simulink model "quadrotor_demo_xpc"  (Simulink 7.4)
settings: Solver=ode4  StartTime=0.0  StopTime=inf  FixedStep=0.01  RelTol=1e-3
libraries: xpcutilitieslib x23, aero_sim_lib x8, xpclib x2, simulink x1
settings Model: Creator=jporter  LastModifiedBy=jporter  SimulationMode=rapid-accelerator
settings SolverCC: AutoInsertRateTranBlk=on
settings DataIOCC: MaxDataPoints=5000  SaveFinalState=on  SaveState=on
settings OptimizationCC: InlineParams=on  EnhancedBackFolding=on  SimCompilerOptimization=On
settings HardwareCC: ProdIntDivRoundTo=Zero  ProdEndianess=LittleEndian  ProdHWDeviceType=Generic->32-bit x86 compatible
settings RTWCC: SystemTargetFile=xpctarget.tlc  TemplateMakefile=xpc_default_tmf  Description=xPC Target  ProcessScript=xpctarget_make_rtw_hook  RTWCompilerOptimization=On
settings xpcTargetCC: TargetFcnLib=ansi_tfl_table_tmw.mat  TargetFunctionLibrary=ANSI_C  ParMdlRefBuildCompliant=off  PortableWordSizes=off  xPCisDownloadable=off  xPCLoadParamSetFile=off

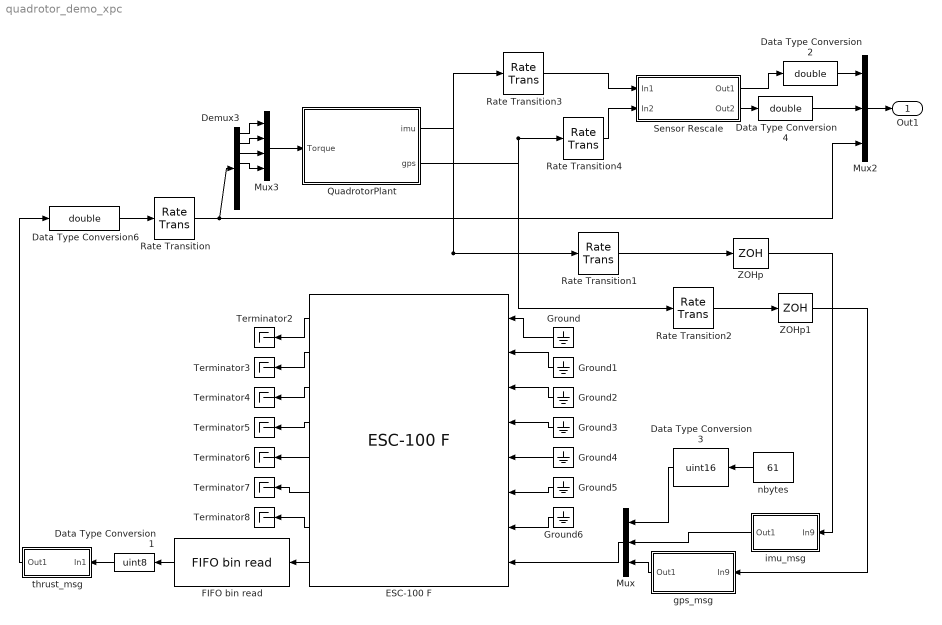
== system quadrotor_demo_xpc ==
  Data Type Conversion1 : DataTypeConversion  OutDataTypeMode=uint8  OutDataType=sfix(16)  OutScaling=2^0  OutDataTypeStr=uint8
  Data Type Conversion2 : DataTypeConversion  OutDataTypeMode=double  OutDataType=sfix(16)  OutScaling=2^0  OutDataTypeStr=double
  Data Type Conversion3 : DataTypeConversion  OutDataTypeMode=uint16  OutDataType=sfix(16)  OutScaling=2^0  OutDataTypeStr=uint16  ConvertRealWorld=Stored Integer (SI)
  Data Type Conversion4 : DataTypeConversion  OutDataTypeMode=double  OutDataType=sfix(16)  OutScaling=2^0  OutDataTypeStr=double
  Data Type Conversion6 : DataTypeConversion  OutDataTypeMode=double  OutDataType=sfix(16)  OutScaling=2^0  OutDataTypeStr=double
  Demux3 : Demux  Outputs=8
  ESC-100 F : xpclib/RS232/Quatech/ESC-100/ESC-100 F  SystemSampleTime=-1  group=Basic Setup  port=8  irqnum=10  slot=-1  baud1=57600  parity1=None  ndata1=8  nstop1=1  fifomode1=64 deep  rlevel1=half full  automode1=off  xmtfifosize1=1024  xmtdatatype1=count+16 bit uint  rcvfifosize1=1024  baud2=57600  parity2=None  ndata2=8  nstop2=1  fifomode2=64 deep  rlevel2=half full  automode2=off  xmtfifosize2=1024  xmtdatatype2=count+16 bit uint  rcvfifosize2=1024  baud3=57600  parity3=None  ndata3=8  nstop3=1  fifomode3=64 deep  rlevel3=half full  automode3=off  xmtfifosize3=1024  xmtdatatype3=count+16 bit uint  rcvfifosize3=1024  buad4=57600  parity4=None  ndata4=8  nstop4=1  fifomode4=64 deep  rlevel4=half full  automode4=off  xmtfifosize4=1024  xmtdatatype4=count+16 bit uint  rcvfifosize4=1024  baud5=57600  parity5=None  ndata5=8  nstop5=1  fifomode5=64 deep  rlevel5=half full  automode5=off  xmtfifosize5=1024  xmtdatatype5=count+16 bit uint  rcvfifosize5=1024  baud6=57600  parity6=None  ndata6=8  nstop6=1  fifomode6=64 deep  rlevel6=half full  automode6=off  xmtfifosize6=1024  xmtdatatype6=count+16 bit uint  rcvfifosize6=1024  baud7=57600  parity7=None  ndata7=8  nstop7=1  fifomode7=64 deep  rlevel7=half full  automode7=off  xmtfifosize7=1024  xmtdatatype7=count+16 bit uint  rcvfifosize7=1024  baud8=57600  parity8=None  ndata8=8  nstop8=1  fifomode8=64 deep  rlevel8=half full  automode8=off  xmtfifosize8=1024  xmtdatatype8=count+16 bit uint  rcvfifosize8=1024
  FIFO bin read : xpclib/RS232/FIFO bin read   header={char([147])}  lengths=[33]  hold=Hold last output if no new data  enable=off  maxsize=33  outputtype=count+16 bit uint  sampletime=-1
  Ground{,1..6} (7 alike) : Ground
  Mux : Mux  Inputs=3
  Mux2 : Mux  Inputs=3
  Mux3 : Mux
  QuadrotorPlant : Subsystem
  Rate Transition : RateTransition
  Rate Transition1 : RateTransition  OutPortSampleTimeOpt=Inherit  OutPortSampleTimeMultiple=2
  Rate Transition2 : RateTransition  OutPortSampleTimeOpt=Inherit  OutPortSampleTimeMultiple=2
  Rate Transition3 : RateTransition
  Rate Transition4 : RateTransition
  Sensor Rescale : Subsystem
  Terminator{2..8} (7 alike) : Terminator
  ZOHp : ZeroOrderHold  SampleTime=0.02
  ZOHp1 : ZeroOrderHold  SampleTime=0.02
  gps_msg : Subsystem
  imu_msg : Subsystem
  nbytes : Constant  Value=61  OutDataTypeMode=uint8  OutDataType=sfix(16)  OutScaling=2^0  OutDataTypeStr=uint8
  thrust_msg : Subsystem
  Out1 : Outport
  wires:
  Rate Transition/1 -> Mux2/3, Demux3/1
  ZOHp/1 -> imu_msg/1(In9)
  Data Type Conversion1/1 -> thrust_msg/1(In1)
  ESC-100 F/1 -> Terminator2/1
  ESC-100 F/2 -> Terminator3/1
  ESC-100 F/3 -> Terminator4/1
  ESC-100 F/4 -> Terminator5/1
  ESC-100 F/5 -> Terminator6/1
  ESC-100 F/6 -> Terminator7/1
  ESC-100 F/7 -> Terminator8/1
  Ground/1 -> ESC-100 F/1
  Ground1/1 -> ESC-100 F/2
  Ground2/1 -> ESC-100 F/3
  Ground3/1 -> ESC-100 F/4
  Ground4/1 -> ESC-100 F/5
  Ground5/1 -> ESC-100 F/6
  ESC-100 F/8 -> FIFO bin read/1
  FIFO bin read/1 -> Data Type Conversion1/1
  Rate Transition1/1 -> ZOHp/1
  Data Type Conversion6/1 -> Rate Transition/1
  thrust_msg/1(Out1) -> Data Type Conversion6/1
  Ground6/1 -> ESC-100 F/7
  Rate Transition2/1 -> ZOHp1/1
  Mux/1 -> ESC-100 F/8
  ZOHp1/1 -> gps_msg/1(In9)
  nbytes/1 -> Data Type Conversion3/1
  imu_msg/1(Out1) -> Mux/2
  gps_msg/1(Out1) -> Mux/3
  Data Type Conversion3/1 -> Mux/1
  QuadrotorPlant/1(imu) -> Rate Transition1/1, Rate Transition3/1
  QuadrotorPlant/2(gps) -> Rate Transition2/1, Rate Transition4/1
  Mux2/1 -> Out1/1
  Data Type Conversion2/1 -> Mux2/1
  Data Type Conversion4/1 -> Mux2/2
  Demux3/1 -> Mux3/1
  Demux3/2 -> Mux3/2
  Demux3/3 -> Mux3/3
  Demux3/4 -> Mux3/4
  Mux3/1 -> QuadrotorPlant/1(Torque)
  Rate Transition3/1 -> Sensor Rescale/1(In1)
  Rate Transition4/1 -> Sensor Rescale/2(In2)
  Sensor Rescale/1(Out1) -> Data Type Conversion2/1
  Sensor Rescale/2(Out2) -> Data Type Conversion4/1

== system quadrotor_demo_xpc/QuadrotorPlant ==
  Torque : Inport
  3DM_GX1 : Subsystem  mask{a_g_s=7000, g_max=5, g_g_s=8500, omega_max=300, Ts=.02}
      mask prompts: a_g_s "AccelGainScale:"; g_max "Max G (1 G = 9.81 m/s^2):"; g_g_s "GyroGainScale:"; omega_max "Mav Angular Velocity (deg/sec):"; Ts "Sample Rate (seconds):"
  Mux : Mux  Inputs=[3 3 3]
  Mux1 : Mux  Inputs=[3 3]
  SUPERSTAR_II : Subsystem  mask{Ts=.2}
      mask prompts: Ts "Sample Rate (seconds):"
  gravity_effects : Constant  Value=zeros(3,1)  OutDataTypeMode=double  OutDataType=sfix(16)  OutScaling=2^0  OutDataTypeStr=double
  starmac_dynamics : Subsystem  AncestorBlock=aero_sim_lib/starmac_dynamics
  imu : Outport
  gps : Outport  Port=2
  wires:
  starmac_dynamics/3(euler) -> 3DM_GX1/1(euler_c)  "euler"
  starmac_dynamics/7(Ab) -> 3DM_GX1/2(Ab_c)
  starmac_dynamics/2(Xe) -> SUPERSTAR_II/1(Xe)  "Xe"
  starmac_dynamics/1(Ve) -> SUPERSTAR_II/2(Ve)  "Ve"
  gravity_effects/1 -> starmac_dynamics/2(wind_velocity)
  starmac_dynamics/5(omega) -> 3DM_GX1/3(omega_c)
  3DM_GX1/1(euler_s) -> Mux/1
  3DM_GX1/2(Ab_s) -> Mux/2
  3DM_GX1/3(omega_s) -> Mux/3
  Mux/1 -> imu/1
  SUPERSTAR_II/1(Xe_s) -> Mux1/1
  SUPERSTAR_II/2(Ve_s) -> Mux1/2
  Mux1/1 -> gps/1
  Torque/1 -> starmac_dynamics/1(desired_motor_thrust)

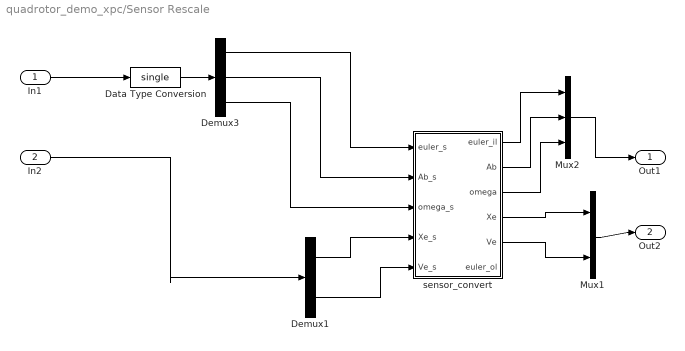
== system quadrotor_demo_xpc/Sensor Rescale ==
  In1 : Inport  OutDataType=fixdt(1, 16)  OutScaling=2^0
  In2 : Inport  Port=2  OutDataType=fixdt(1, 16)  OutScaling=2^0
  Data Type Conversion : DataTypeConversion  OutDataTypeMode=single  OutDataType=fixdt(1, 16)  OutScaling=2^0  OutDataTypeStr=single
  Demux1 : Demux  Outputs=[3 3]
  Demux3 : Demux  Outputs=[3 3 3]
  Mux1 : Mux  Inputs=2
  Mux2 : Mux  Inputs=3
  sensor_convert : Subsystem  mask{a_g_s=7000, g_g_s=8500}
      mask prompts: a_g_s "AccelGainScale[a_g_s]:"; g_g_s "GyroGainScale[g_g_s]:"
  Out1 : Outport  OutDataType=fixdt(1, 16)  OutScaling=2^0
  Out2 : Outport  Port=2  OutDataType=fixdt(1, 16)  OutScaling=2^0
  wires:
  sensor_convert/1(euler_il) -> Mux2/1
  sensor_convert/2(Ab) -> Mux2/2
  sensor_convert/3(omega) -> Mux2/3
  Mux2/1 -> Out1/1
  sensor_convert/4(Xe) -> Mux1/1
  sensor_convert/5(Ve) -> Mux1/2
  Mux1/1 -> Out2/1
  Data Type Conversion/1 -> Demux3/1
  In1/1 -> Data Type Conversion/1
  Demux3/1 -> sensor_convert/1(euler_s)
  Demux3/2 -> sensor_convert/2(Ab_s)
  Demux3/3 -> sensor_convert/3(omega_s)
  Demux1/1 -> sensor_convert/4(Xe_s)
  Demux1/2 -> sensor_convert/5(Ve_s)
  In2/1 -> Demux1/1

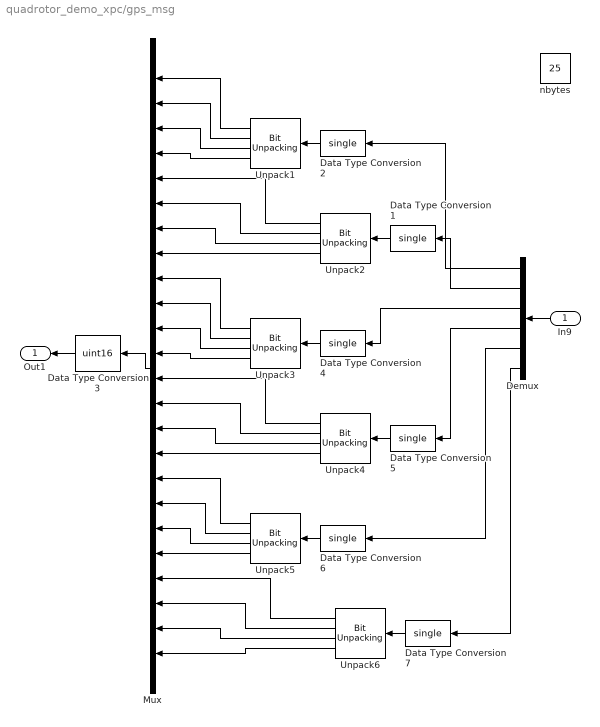
== system quadrotor_demo_xpc/gps_msg ==
  In9 : Inport
  Data Type Conversion{1..2,4..7} (6 alike) : DataTypeConversion  OutDataTypeMode=single  OutDataType=sfix(16)  OutScaling=2^0  OutDataTypeStr=single
  Data Type Conversion3 : DataTypeConversion  OutDataTypeMode=uint16  OutDataType=sfix(16)  OutScaling=2^0  OutDataTypeStr=uint16  ConvertRealWorld=Stored Integer (SI)
  Demux : Demux  Outputs=6
  Mux : Mux  Inputs=24
  Unpack{1..6} (6 alike) : xpcutilitieslib/Bit Unpacking   SignExtend=off  MaskBitPatterns={[0:7], [8:15], [16:23], [24:31]}  MaskPackDataType=single  MaskPackDataSize=[1]  MaskUnpackDataTypes={'uint8', 'uint8', 'uint8', 'uint8'}  MaskUnpackDataSizes={[1], [1], [1], [1]}
  nbytes : Constant  Value=25  OutDataTypeMode=uint8  OutDataType=sfix(16)  OutScaling=2^0  OutDataTypeStr=uint8
  Out1 : Outport
  wires:
  Mux/1 -> Data Type Conversion3/1
  Data Type Conversion2/1 -> Unpack1/1
  Data Type Conversion3/1 -> Out1/1
  Data Type Conversion1/1 -> Unpack2/1
  Data Type Conversion4/1 -> Unpack3/1
  Data Type Conversion5/1 -> Unpack4/1
  Data Type Conversion6/1 -> Unpack5/1
  Data Type Conversion7/1 -> Unpack6/1
  In9/1 -> Demux/1
  Demux/1 -> Data Type Conversion2/1
  Demux/2 -> Data Type Conversion1/1
  Demux/3 -> Data Type Conversion4/1
  Demux/4 -> Data Type Conversion5/1
  Demux/5 -> Data Type Conversion6/1
  Demux/6 -> Data Type Conversion7/1
  Unpack1/1 -> Mux/1
  Unpack1/2 -> Mux/2
  Unpack1/3 -> Mux/3
  Unpack1/4 -> Mux/4
  Unpack2/1 -> Mux/5
  Unpack2/2 -> Mux/6
  Unpack2/3 -> Mux/7
  Unpack2/4 -> Mux/8
  Unpack3/1 -> Mux/9
  Unpack3/2 -> Mux/10
  Unpack3/3 -> Mux/11
  Unpack3/4 -> Mux/12
  Unpack4/1 -> Mux/13
  Unpack4/2 -> Mux/14
  Unpack4/3 -> Mux/15
  Unpack4/4 -> Mux/16
  Unpack5/1 -> Mux/17
  Unpack5/2 -> Mux/18
  Unpack5/3 -> Mux/19
  Unpack5/4 -> Mux/20
  Unpack6/1 -> Mux/21
  Unpack6/2 -> Mux/22
  Unpack6/3 -> Mux/23
  Unpack6/4 -> Mux/24

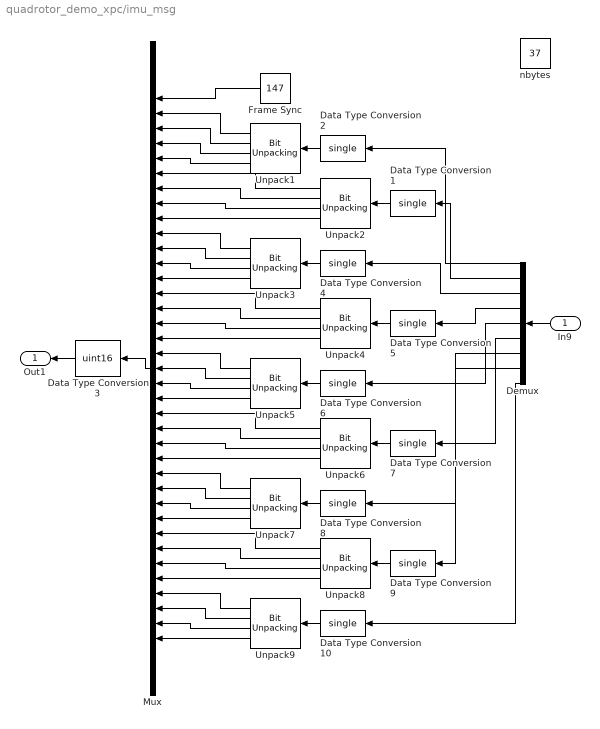
== system quadrotor_demo_xpc/imu_msg ==
  In9 : Inport
  Data Type Conversion{1..2,4..10} (9 alike) : DataTypeConversion  OutDataTypeMode=single  OutDataType=sfix(16)  OutScaling=2^0  OutDataTypeStr=single
  Data Type Conversion3 : DataTypeConversion  OutDataTypeMode=uint16  OutDataType=sfix(16)  OutScaling=2^0  OutDataTypeStr=uint16  ConvertRealWorld=Stored Integer (SI)
  Demux : Demux  Outputs=9
  Frame Sync : Constant  Value=147  OutDataTypeMode=uint8  OutDataType=sfix(16)  OutScaling=2^0  OutDataTypeStr=uint8
  Mux : Mux  Inputs=37
  Unpack{1..9} (9 alike) : xpcutilitieslib/Bit Unpacking   SignExtend=off  MaskBitPatterns={[0:7], [8:15], [16:23], [24:31]}  MaskPackDataType=single  MaskPackDataSize=[1]  MaskUnpackDataTypes={'uint8', 'uint8', 'uint8', 'uint8'}  MaskUnpackDataSizes={[1], [1], [1], [1]}
  nbytes : Constant  Value=37  OutDataTypeMode=uint8  OutDataType=sfix(16)  OutScaling=2^0  OutDataTypeStr=uint8
  Out1 : Outport
  wires:
  Mux/1 -> Data Type Conversion3/1
  Data Type Conversion2/1 -> Unpack1/1
  Data Type Conversion3/1 -> Out1/1
  Data Type Conversion1/1 -> Unpack2/1
  Data Type Conversion4/1 -> Unpack3/1
  Data Type Conversion5/1 -> Unpack4/1
  Data Type Conversion6/1 -> Unpack5/1
  Data Type Conversion7/1 -> Unpack6/1
  Data Type Conversion8/1 -> Unpack7/1
  Data Type Conversion9/1 -> Unpack8/1
  Data Type Conversion10/1 -> Unpack9/1
  In9/1 -> Demux/1
  Demux/1 -> Data Type Conversion2/1
  Demux/2 -> Data Type Conversion1/1
  Demux/3 -> Data Type Conversion4/1
  Demux/4 -> Data Type Conversion5/1
  Demux/5 -> Data Type Conversion6/1
  Demux/6 -> Data Type Conversion7/1
  Demux/7 -> Data Type Conversion8/1
  Demux/8 -> Data Type Conversion9/1
  Demux/9 -> Data Type Conversion10/1
  Frame Sync/1 -> Mux/1
  Unpack1/1 -> Mux/2
  Unpack1/2 -> Mux/3
  Unpack1/3 -> Mux/4
  Unpack1/4 -> Mux/5
  Unpack2/1 -> Mux/6
  Unpack2/2 -> Mux/7
  Unpack2/3 -> Mux/8
  Unpack2/4 -> Mux/9
  Unpack3/1 -> Mux/10
  Unpack3/2 -> Mux/11
  Unpack3/3 -> Mux/12
  Unpack3/4 -> Mux/13
  Unpack4/1 -> Mux/14
  Unpack4/2 -> Mux/15
  Unpack4/3 -> Mux/16
  Unpack4/4 -> Mux/17
  Unpack5/1 -> Mux/18
  Unpack5/2 -> Mux/19
  Unpack5/3 -> Mux/20
  Unpack5/4 -> Mux/21
  Unpack6/1 -> Mux/22
  Unpack6/2 -> Mux/23
  Unpack6/3 -> Mux/24
  Unpack6/4 -> Mux/25
  Unpack7/1 -> Mux/26
  Unpack7/2 -> Mux/27
  Unpack7/3 -> Mux/28
  Unpack7/4 -> Mux/29
  Unpack8/1 -> Mux/30
  Unpack8/2 -> Mux/31
  Unpack8/3 -> Mux/32
  Unpack8/4 -> Mux/33
  Unpack9/1 -> Mux/34
  Unpack9/2 -> Mux/35
  Unpack9/3 -> Mux/36
  Unpack9/4 -> Mux/37

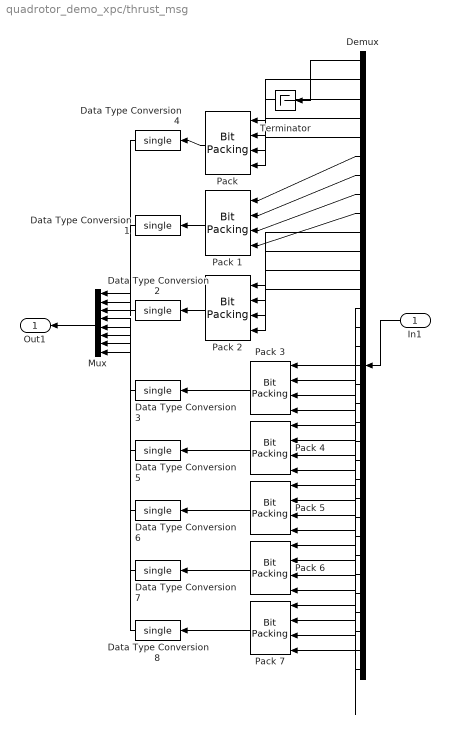
== system quadrotor_demo_xpc/thrust_msg ==
  In1 : Inport
  Data Type Conversion{1..8} (8 alike) : DataTypeConversion  OutDataTypeMode=single  OutDataType=sfix(16)  OutScaling=2^0  OutDataTypeStr=single
  Demux : Demux  Outputs=33
  Mux : Mux  Inputs=8
  Pack {,1..7} (8 alike) : xpcutilitieslib/Bit Packing   MaskBitPatterns={[0:7], [8:15], [16:23], [24:31]}  MaskPackDataType=single  MaskPackDataSize=[1]
  Terminator : Terminator
  Out1 : Outport
  wires:
  Demux/1 -> Terminator/1
  "Pack "/1 -> Data Type Conversion4/1
  Demux/2 -> "Pack "/1
  Demux/3 -> "Pack "/2
  Demux/4 -> "Pack "/3
  Demux/5 -> "Pack "/4
  In1/1 -> Demux/1
  Pack 1/1 -> Data Type Conversion1/1
  Demux/6 -> Pack 1/1
  Demux/7 -> Pack 1/2
  Demux/8 -> Pack 1/3
  Demux/9 -> Pack 1/4
  Pack 2/1 -> Data Type Conversion2/1
  Demux/10 -> Pack 2/1
  Demux/11 -> Pack 2/2
  Demux/12 -> Pack 2/3
  Demux/13 -> Pack 2/4
  Pack 3/1 -> Data Type Conversion3/1
  Demux/14 -> Pack 3/1
  Demux/15 -> Pack 3/2
  Demux/16 -> Pack 3/3
  Demux/17 -> Pack 3/4
  Data Type Conversion4/1 -> Mux/1
  Mux/1 -> Out1/1
  Data Type Conversion1/1 -> Mux/2
  Data Type Conversion2/1 -> Mux/3
  Data Type Conversion3/1 -> Mux/4
  Pack 4/1 -> Data Type Conversion5/1
  Pack 5/1 -> Data Type Conversion6/1
  Pack 6/1 -> Data Type Conversion7/1
  Pack 7/1 -> Data Type Conversion8/1
  Demux/18 -> Pack 4/1
  Demux/19 -> Pack 4/2
  Demux/20 -> Pack 4/3
  Demux/21 -> Pack 4/4
  Demux/22 -> Pack 5/1
  Demux/23 -> Pack 5/2
  Demux/24 -> Pack 5/3
  Demux/25 -> Pack 5/4
  Demux/26 -> Pack 6/1
  Demux/27 -> Pack 6/2
  Demux/28 -> Pack 6/3
  Demux/29 -> Pack 6/4
  Demux/30 -> Pack 7/1
  Demux/31 -> Pack 7/2
  Demux/32 -> Pack 7/3
  Demux/33 -> Pack 7/4
  Data Type Conversion5/1 -> Mux/5
  Data Type Conversion6/1 -> Mux/6
  Data Type Conversion7/1 -> Mux/7
  Data Type Conversion8/1 -> Mux/8

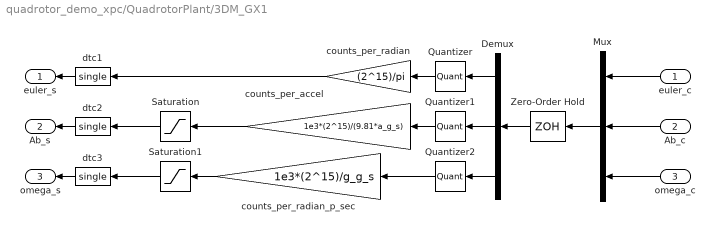
== system quadrotor_demo_xpc/QuadrotorPlant/3DM_GX1 ==
  euler_c : Inport
  Ab_c : Inport  Port=2
  omega_c : Inport  Port=3
  Demux : Demux  Outputs=[3 3 3]
  Mux : Mux  Inputs=[3 3 3]
  Quantizer : Quantizer  QuantizationInterval=pi/(2^15)*ones(3,1)
  Quantizer1 : Quantizer  QuantizationInterval=g_max*9.81/(2^15)*ones(3,1)
  Quantizer2 : Quantizer  QuantizationInterval=(pi*omega_max/180)/(2^15)*ones(3,1)
  Saturation : Saturate  UpperLimit=((2^15)-1)*ones(3,1)  LowerLimit=-(2^15)*ones(3,1)  OutDataType=sfix(16)  OutScaling=2^0
  Saturation1 : Saturate  UpperLimit=((2^15)-1)*ones(3,1)  LowerLimit=-(2^15)*ones(3,1)  OutDataType=sfix(16)  OutScaling=2^0
  Zero-Order Hold : ZeroOrderHold  SampleTime=Ts
  counts_per_accel : Gain  Gain=1e3*(2^15)/(9.81*a_g_s)  ParameterDataType=sfix(16)  ParameterScaling=2^0  OutDataType=sfix(16)  OutScaling=2^0
  counts_per_radian : Gain  Gain=(2^15)/pi  ParameterDataType=sfix(16)  ParameterScaling=2^0  OutDataType=sfix(16)  OutScaling=2^0
  counts_per_radian_p_sec : Gain  Gain=1e3*(2^15)/g_g_s  ParameterDataType=sfix(16)  ParameterScaling=2^0  OutDataType=sfix(16)  OutScaling=2^0
  dtc1 : DataTypeConversion  OutDataTypeMode=single  OutDataType=sfix(16)  OutScaling=2^0  OutDataTypeStr=single
  dtc2 : DataTypeConversion  OutDataTypeMode=single  OutDataType=sfix(16)  OutScaling=2^0  OutDataTypeStr=single
  dtc3 : DataTypeConversion  OutDataTypeMode=single  OutDataType=sfix(16)  OutScaling=2^0  OutDataTypeStr=single
  euler_s : Outport
  Ab_s : Outport  Port=2
  omega_s : Outport  Port=3
  wires:
  Mux/1 -> Zero-Order Hold/1
  euler_c/1 -> Mux/1
  Ab_c/1 -> Mux/2
  omega_c/1 -> Mux/3
  Zero-Order Hold/1 -> Demux/1
  Demux/1 -> Quantizer/1
  Demux/2 -> Quantizer1/1
  Quantizer/1 -> counts_per_radian/1
  Quantizer1/1 -> counts_per_accel/1
  counts_per_accel/1 -> Saturation/1
  Demux/3 -> Quantizer2/1
  counts_per_radian_p_sec/1 -> Saturation1/1
  Quantizer2/1 -> counts_per_radian_p_sec/1
  Saturation/1 -> dtc2/1
  Saturation1/1 -> dtc3/1
  dtc1/1 -> euler_s/1
  dtc2/1 -> Ab_s/1
  dtc3/1 -> omega_s/1
  counts_per_radian/1 -> dtc1/1

== system quadrotor_demo_xpc/QuadrotorPlant/SUPERSTAR_II ==
  Xe : Inport
  Ve : Inport  Port=2
  Demux : Demux  Outputs=[3 3]
  Mux : Mux  Inputs=[3 3]
  Rate Transition : RateTransition
  ZOH : ZeroOrderHold  SampleTime=Ts
  dtc1 : DataTypeConversion  OutDataTypeMode=single  OutDataType=sfix(16)  OutScaling=2^0  OutDataTypeStr=single
  dtc2 : DataTypeConversion  OutDataTypeMode=single  OutDataType=sfix(16)  OutScaling=2^0  OutDataTypeStr=single
  Xe_s : Outport
  Ve_s : Outport  Port=2
  wires:
  ZOH/1 -> Rate Transition/1
  Ve/1 -> Mux/2
  Xe/1 -> Mux/1
  Mux/1 -> ZOH/1
  Demux/1 -> dtc1/1
  Demux/2 -> dtc2/1
  dtc1/1 -> Xe_s/1
  dtc2/1 -> Ve_s/1
  Rate Transition/1 -> Demux/1

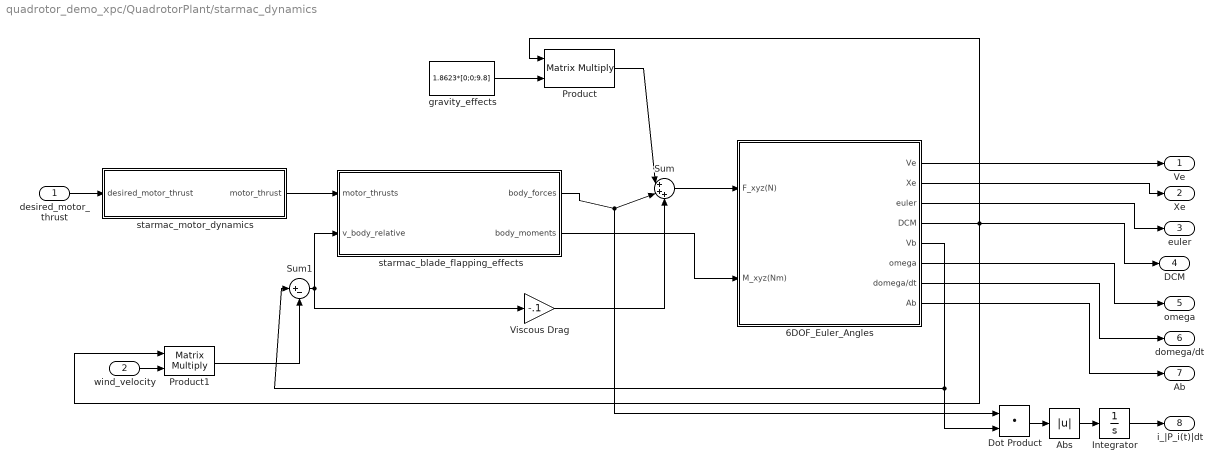
== system quadrotor_demo_xpc/QuadrotorPlant/starmac_dynamics ==
  desired_motor_thrust : Inport  OutDataType=sfix(16)  OutScaling=2^0
  wind_velocity : Inport  Port=2  OutDataType=sfix(16)  OutScaling=2^0
  6DOF_Euler_Angles : Subsystem  AncestorBlock=aero_sim_lib/6DOF (Euler Angles)_CMU  mask{XYZe_0=[0.1;0.2;0], Vb_0=[0;0;0], euler_0=[0;0;0], omega_0=[0;0;0], M=1.8623, I=diag([0.02759 0.02771 0.04806])}
      mask prompts: XYZe_0 "Initial position in inertial axes [Xe,Ye,Ze]:"; Vb_0 "Initial velocity in body axes [U,v,w]:"; euler_0 "Initial Euler orientation [roll, pitch, yaw]=[phi,theta,psi]:"; omega_0 "Initial body rotation rates [p,q,r]=omega:"; M "Initial mass:"; I "Inertial:"
  Abs : Abs  OutDataType=sfix(16)  OutScaling=2^0
  Dot Product : DotProduct  OutDataType=sfix(16)  OutScaling=2^-10  InputSameDT=on  OutDataTypeStr=Inherit: Inherit via internal rule
  Integrator : Integrator
  Product : Product  Multiplication=Matrix(*)  OutDataType=sfix(16)  OutScaling=2^0  RndMeth=Zero
  Product1 : Product  Multiplication=Matrix(*)  OutDataType=sfix(16)  OutScaling=2^0  RndMeth=Zero
  Sum : Sum  Inputs=|+++  OutDataType=sfix(16)  OutScaling=2^0
  Sum1 : Sum  Inputs=|+-  OutDataType=sfix(16)  OutScaling=2^0
  Viscous Drag : Gain  Gain=-.1  ParameterDataType=sfix(16)  ParameterScaling=2^0  OutDataType=sfix(16)  OutScaling=2^0
  gravity_effects : Constant  Value=1.8623*[0;0;9.8]  OutDataType=sfix(16)  OutScaling=2^0
  starmac_blade_flapping_effects : Subsystem  AncestorBlock=aero_sim_lib/starmac_blade_flapping_effects
  starmac_motor_dynamics : Subsystem  AncestorBlock=aero_sim_lib/starmac_motor_dynamics  mask{tau_motor=.1, T_nom=1.8263*9.8/4, thrust_max=9.8, thrust_min=0, motor_lag_enable=on, motor_variance=.01*(.05*9.8/4)^2, Ts=1/50}
      mask prompts: tau_motor "tau_motor (seconds):"; T_nom "nominal thrust (N):"; thrust_max "maximum thrust (N):"; thrust_min "minimum thrust (N):"; motor_lag_enable "Motor Lag Enabled:"; motor_variance "Motor Variance [motor_variance]:"; Ts "Motor Update Rate (seconds):"
  Ve : Outport  OutDataType=sfix(16)  OutScaling=2^0
  Xe : Outport  Port=2  OutDataType=sfix(16)  OutScaling=2^0
  euler : Outport  Port=3  OutDataType=sfix(16)  OutScaling=2^0
  DCM : Outport  Port=4  OutDataType=sfix(16)  OutScaling=2^0
  omega : Outport  Port=5  OutDataType=sfix(16)  OutScaling=2^0
  domega/dt : Outport  Port=6  OutDataType=sfix(16)  OutScaling=2^0
  Ab : Outport  Port=7  OutDataType=sfix(16)  OutScaling=2^0
  i_|P_i(t)|dt : Outport  Port=8  OutDataType=sfix(16)  OutScaling=2^0
  wires:
  wind_velocity/1 -> Product1/2
  desired_motor_thrust/1 -> starmac_motor_dynamics/1(desired_motor_thrust)
  starmac_blade_flapping_effects/1(body_forces) -> Sum/2, Dot Product/1
  starmac_blade_flapping_effects/2(body_moments) -> 6DOF_Euler_Angles/2(M_xyz(Nm))
  Viscous Drag/1 -> Sum/3
  6DOF_Euler_Angles/5(Vb) -> Sum1/1, Dot Product/2
  Product1/1 -> Sum1/2
  Sum1/1 -> Viscous Drag/1, starmac_blade_flapping_effects/2(v_body_relative)
  gravity_effects/1 -> Product/2
  6DOF_Euler_Angles/4(DCM) -> Product1/1, Product/1, DCM/1
  Sum/1 -> 6DOF_Euler_Angles/1(F_xyz(N))
  Product/1 -> Sum/1
  starmac_motor_dynamics/1(motor_thrust) -> starmac_blade_flapping_effects/1(motor_thrusts)
  6DOF_Euler_Angles/1(Ve) -> Ve/1
  6DOF_Euler_Angles/2(Xe) -> Xe/1
  6DOF_Euler_Angles/3(euler) -> euler/1
  6DOF_Euler_Angles/6(omega) -> omega/1
  6DOF_Euler_Angles/7(domega/dt) -> domega/dt/1
  6DOF_Euler_Angles/8(Ab) -> Ab/1
  Integrator/1 -> i_|P_i(t)|dt/1
  Dot Product/1 -> Abs/1
  Abs/1 -> Integrator/1

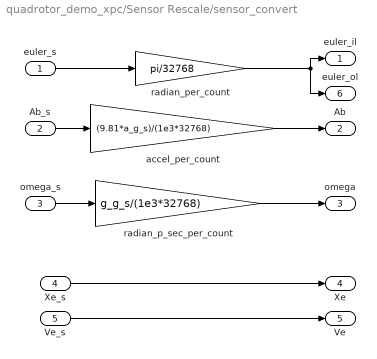
== system quadrotor_demo_xpc/Sensor Rescale/sensor_convert ==
  euler_s : Inport  PortDimensions=[3]
  Ab_s : Inport  Port=2  PortDimensions=[3]
  omega_s : Inport  Port=3  PortDimensions=[3]
  Xe_s : Inport  Port=4  PortDimensions=[3]  DataType=single  OutDataTypeStr=single
  Ve_s : Inport  Port=5  PortDimensions=[3]  DataType=single  OutDataTypeStr=single
  accel_per_count : Gain  Gain=(9.81*a_g_s)/(1e3*32768)  ParameterDataTypeMode=single  ParameterDataType=sfix(16)  ParameterScaling=2^0  ParamDataTypeStr=single  OutDataTypeMode=single  OutDataType=sfix(16)  OutScaling=2^0  OutDataTypeStr=single
  radian_p_sec_per_count : Gain  Gain=g_g_s/(1e3*32768)  ParameterDataTypeMode=single  ParameterDataType=sfix(16)  ParameterScaling=2^0  ParamDataTypeStr=single  OutDataTypeMode=single  OutDataType=sfix(16)  OutScaling=2^0  OutDataTypeStr=single
  radian_per_count : Gain  Gain=pi/32768  ParameterDataTypeMode=single  ParameterDataType=sfix(16)  ParameterScaling=2^0  ParamDataTypeStr=single  OutDataTypeMode=single  OutDataType=sfix(16)  OutScaling=2^0  OutDataTypeStr=single
  euler_il : Outport
  Ab : Outport  Port=2
  omega : Outport  Port=3
  Xe : Outport  Port=4
  Ve : Outport  Port=5
  euler_ol : Outport  Port=6
  wires:
  euler_s/1 -> radian_per_count/1
  radian_per_count/1 -> euler_il/1, euler_ol/1
  Ab_s/1 -> accel_per_count/1
  accel_per_count/1 -> Ab/1
  omega_s/1 -> radian_p_sec_per_count/1
  radian_p_sec_per_count/1 -> omega/1
  Xe_s/1 -> Xe/1
  Ve_s/1 -> Ve/1

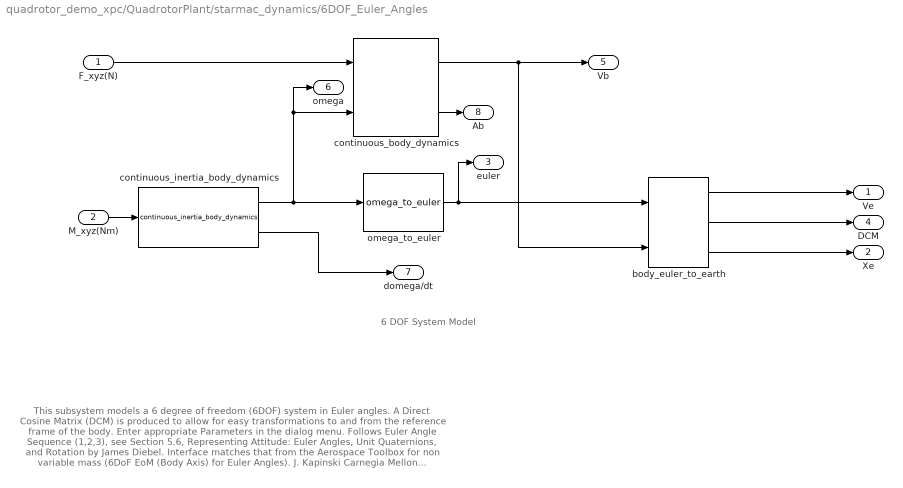
== system quadrotor_demo_xpc/QuadrotorPlant/starmac_dynamics/6DOF_Euler_Angles ==
  note: This subsystem models a 6 degree of freedom (6DOF) system in Euler angles.
      | A Direct Cosine Matrix (DCM) is produced to allow for easy transformations to
      | and from the reference frame of the body.  Enter appropriate Parameters in the dialog menu.
      | Follows Euler Angle Sequence (1,2,3), see Section 5.6, Representing Attitude: Euler Angles, Unit
      | Quaternions, and Rotation by James Diebel.  Interface matches that from the Aerospace Toolbox
      | for non variable mass (6DoF EoM (Body Axis) for Euler Angles).
      |
      | J. Kapinski
      | Carnegia Mellon University
      | 7/2007
      | Revised:
      | Nicholas Kottenstette, ISIS, 8/2008
  note: 6 DOF System Model
  F_xyz(N) : Inport  OutDataType=sfix(16)  OutScaling=2^0
  M_xyz(Nm) : Inport  Port=2  PortDimensions=3  OutDataType=sfix(16)  OutScaling=2^0
  body_euler_to_earth : aero_sim_lib/body_euler_to_earth  SystemSampleTime=-1  XYZe_0=XYZe_0
  continuous_body_dynamics : aero_sim_lib/continuous_body_dynamics  SystemSampleTime=-1  M=M  Vb_0=Vb_0
  continuous_inertia_body_dynamics : aero_sim_lib/continuous_inertia_body_dynamics  SystemSampleTime=-1  I=I  omega_0=omega_0
  omega_to_euler : aero_sim_lib/omega_to_euler  SystemSampleTime=-1  euler_0=euler_0
  Ve : Outport  OutDataType=sfix(16)  OutScaling=2^0
  Xe : Outport  Port=2  OutDataType=sfix(16)  OutScaling=2^0
  euler : Outport  Port=3  OutDataType=sfix(16)  OutScaling=2^0
  DCM : Outport  Port=4  OutDataType=sfix(16)  OutScaling=2^0
  Vb : Outport  Port=5  OutDataType=sfix(16)  OutScaling=2^0
  omega : Outport  Port=6  OutDataType=sfix(16)  OutScaling=2^0
  domega/dt : Outport  Port=7  OutDataType=sfix(16)  OutScaling=2^0
  Ab : Outport  Port=8  OutDataType=sfix(16)  OutScaling=2^0
  wires:
  body_euler_to_earth/3 -> Xe/1
  body_euler_to_earth/2 -> DCM/1
  body_euler_to_earth/1 -> Ve/1
  omega_to_euler/1 -> body_euler_to_earth/1, euler/1
  continuous_inertia_body_dynamics/2 -> domega/dt/1
  continuous_body_dynamics/2 -> Ab/1
  continuous_body_dynamics/1 -> body_euler_to_earth/2, Vb/1
  continuous_inertia_body_dynamics/1 -> omega_to_euler/1, continuous_body_dynamics/2, omega/1
  F_xyz(N)/1 -> continuous_body_dynamics/1
  M_xyz(Nm)/1 -> continuous_inertia_body_dynamics/1

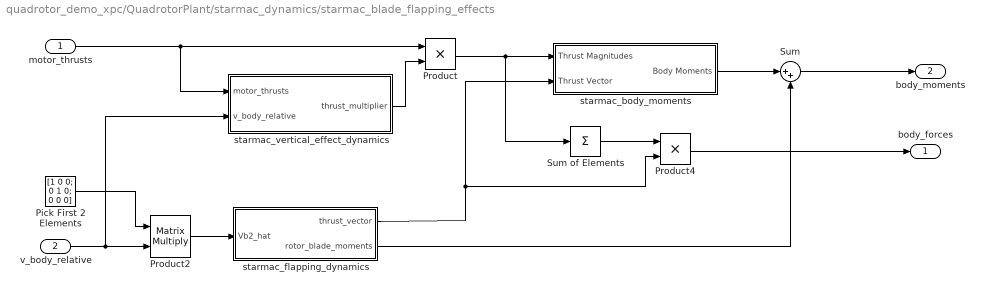
== system quadrotor_demo_xpc/QuadrotorPlant/starmac_dynamics/starmac_blade_flapping_effects ==
  motor_thrusts : Inport  OutDataType=sfix(16)  OutScaling=2^0
  v_body_relative : Inport  Port=2  OutDataType=sfix(16)  OutScaling=2^0
  Pick First 2 Elements : Constant  Value=[1 0 0; 0 1 0; 0 0 0]  OutDataType=sfix(16)  OutScaling=2^0
  Product : Product  OutDataType=sfix(16)  OutScaling=2^0  RndMeth=Zero
  Product2 : Product  Multiplication=Matrix(*)  OutDataType=sfix(16)  OutScaling=2^0  RndMeth=Zero
  Product4 : Product  OutDataType=sfix(16)  OutScaling=2^0  RndMeth=Zero
  Sum : Sum  Inputs=|++  OutDataType=sfix(16)  OutScaling=2^0
  Sum of Elements : Sum  Inputs=+  OutDataType=sfix(16)  OutScaling=2^-10
  starmac_body_moments : Subsystem  AncestorBlock=aero_sim_lib/starmac_body_moments  mask{dx=.3048, dz=.07, K_torque=.47}
  starmac_flapping_dynamics : Subsystem  AncestorBlock=aero_sim_lib/starmac_flapping_dynamics  mask{K_a1s=.009, K_beta=.23}
  starmac_vertical_effect_dynamics : Subsystem  AncestorBlock=aero_sim_lib/starmac_vertical_effect_dynamics  mask{tau_motor=0.1, R=0.127, Alpha=(pi/180)*[-85:5:85], Vinf=[0:0.5:6], Thrust=9.8*[0.3:0.02:0.8]}
      mask prompts: tau_motor "motor time constant (s)"; R "radius of propeller (m)"; Alpha "Alpha (radians)"; Vinf "Vinf (radians)"; Thrust "Propeller Thrust (N)"
      mask init:
      | rho = 1.2;
      | A = pi*R^2;
      | Vh = sqrt(Thrust/(2*rho*A));
      | for i = 1:length(Vh)
      |     for j = 1:length(Vinf)
      |         for k = 1:length(Alpha)
      |             Vi(k,j,i) = find_vi(Vh(i),Vinf(j),Alpha(k));
      |             ToverTh(k,j,i) = min(10,max(0.1,Vh(i)/(Vi(k,j,i)+Vinf(j)*sin(Alpha(k)))));
      |         end
      |     end
      | end
  body_forces : Outport  OutDataType=sfix(16)  OutScaling=2^0
  body_moments : Outport  Port=2  OutDataType=sfix(16)  OutScaling=2^0
  wires:
  starmac_flapping_dynamics/2(rotor_blade_moments) -> Sum/2
  Sum/1 -> body_moments/1
  starmac_body_moments/1(Body Moments) -> Sum/1
  starmac_flapping_dynamics/1(thrust_vector) -> Product4/2, starmac_body_moments/2(Thrust Vector)
  Product4/1 -> body_forces/1
  Sum of Elements/1 -> Product4/1
  Product2/1 -> starmac_flapping_dynamics/1(Vb2_hat)
  v_body_relative/1 -> Product2/2, starmac_vertical_effect_dynamics/2(v_body_relative)
  Pick First 2 Elements/1 -> Product2/1
  motor_thrusts/1 -> Product/1, starmac_vertical_effect_dynamics/1(motor_thrusts)
  starmac_vertical_effect_dynamics/1(thrust_multiplier) -> Product/2
  Product/1 -> Sum of Elements/1, starmac_body_moments/1(Thrust Magnitudes)

== system quadrotor_demo_xpc/QuadrotorPlant/starmac_dynamics/starmac_motor_dynamics ==
  desired_motor_thrust : Inport  OutDataType=sfix(16)  OutScaling=2^0
  Band-Limited White Noise : simulink/Sources/Band-Limited White Noise  SystemSampleTime=-1  Cov=Ts*motor_variance*ones(4,1)  Ts=Ts  seed=22341+[0 1 2 3]'
  Constant : Constant  Value=motor_lag_enable  OutDataType=sfix(16)  OutScaling=2^0
  Saturation : Saturate  UpperLimit=thrust_max*ones(4,1)  LowerLimit=thrust_min*ones(4,1)
  State-Space : StateSpace  A=-(1/tau_motor)*eye(4)  B=(1/tau_motor)*eye(4)  C=eye(4)  D=zeros(4,4)  X0=T_nom*ones(4,1)
  Sum : Sum  Inputs=|++  OutDataType=sfix(16)  OutScaling=2^0
  Switch : Switch  Criteria=u2 > Threshold  OutDataType=sfix(16)  OutScaling=2^0
  motor_thrust : Outport  OutDataType=sfix(16)  OutScaling=2^0
  wires:
  desired_motor_thrust/1 -> State-Space/1, Switch/3
  Sum/1 -> motor_thrust/1
  Saturation/1 -> Sum/1
  Band-Limited White Noise/1 -> Sum/2
  State-Space/1 -> Switch/1
  Switch/1 -> Saturation/1
  Constant/1 -> Switch/2

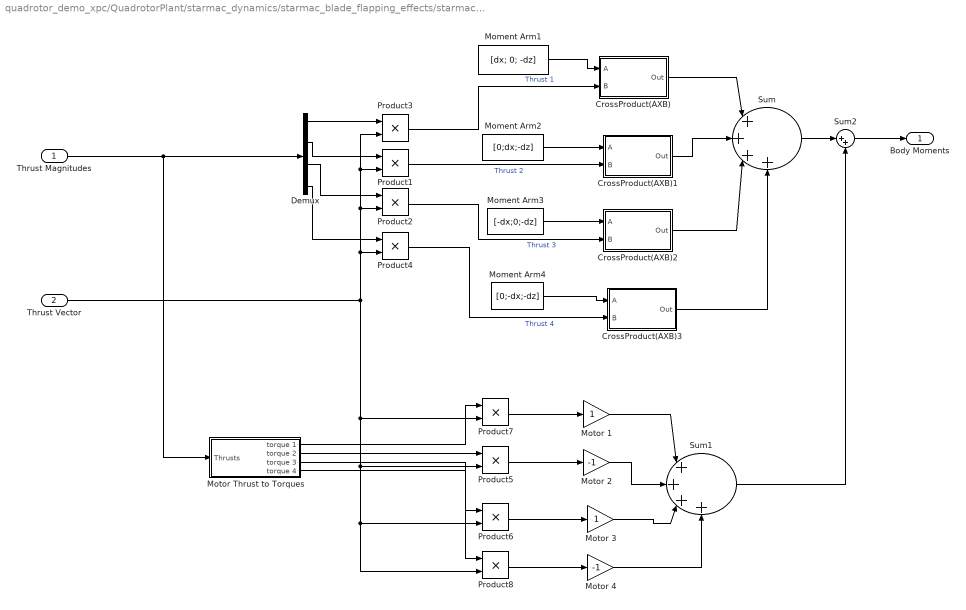
== system quadrotor_demo_xpc/QuadrotorPlant/starmac_dynamics/starmac_blade_flapping_effects/starmac_body_moments ==
  Thrust Magnitudes : Inport  OutDataType=sfix(16)  OutScaling=2^0
  Thrust Vector : Inport  Port=2  OutDataType=sfix(16)  OutScaling=2^0
  CrossProduct(AXB) : Subsystem
  CrossProduct(AXB)1 : Subsystem
  CrossProduct(AXB)2 : Subsystem
  CrossProduct(AXB)3 : Subsystem
  Demux : Demux
  Moment Arm1 : Constant  Value=[dx; 0; -dz]  OutDataType=sfix(16)  OutScaling=2^0
  Moment Arm2 : Constant  Value=[0;dx;-dz]  OutDataType=sfix(16)  OutScaling=2^0
  Moment Arm3 : Constant  Value=[-dx;0;-dz]  OutDataType=sfix(16)  OutScaling=2^0
  Moment Arm4 : Constant  Value=[0;-dx;-dz]  OutDataType=sfix(16)  OutScaling=2^0
  Motor 1 : Gain  ParameterDataType=sfix(16)  ParameterScaling=2^0  OutDataType=sfix(16)  OutScaling=2^0
  Motor 2 : Gain  Gain=-1  ParameterDataType=sfix(16)  ParameterScaling=2^0  OutDataType=sfix(16)  OutScaling=2^0
  Motor 3 : Gain  ParameterDataType=sfix(16)  ParameterScaling=2^0  OutDataType=sfix(16)  OutScaling=2^0
  Motor 4 : Gain  Gain=-1  ParameterDataType=sfix(16)  ParameterScaling=2^0  OutDataType=sfix(16)  OutScaling=2^0
  Motor Thrust to Torques : Subsystem
  Product{1..8} (8 alike) : Product  OutDataType=sfix(16)  OutScaling=2^0  RndMeth=Zero
  Sum : Sum  Inputs=|++++  OutDataType=sfix(16)  OutScaling=2^0
  Sum1 : Sum  Inputs=|++++  OutDataType=sfix(16)  OutScaling=2^0
  Sum2 : Sum  Inputs=|++  OutDataType=sfix(16)  OutScaling=2^0
  Body Moments : Outport  OutDataType=sfix(16)  OutScaling=2^0
  wires:
  CrossProduct(AXB)1/1(Out) -> Sum/2
  Motor Thrust to Torques/4(torque 4) -> Product8/1
  Motor Thrust to Torques/3(torque 3) -> Product6/1
  Motor Thrust to Torques/2(torque 2) -> Product5/1
  Motor Thrust to Torques/1(torque 1) -> Product7/1
  Product8/1 -> Motor 4/1
  Product6/1 -> Motor 3/1
  Product5/1 -> Motor 2/1
  Product7/1 -> Motor 1/1
  Sum2/1 -> Body Moments/1
  Sum1/1 -> Sum2/2
  Sum/1 -> Sum2/1
  Motor 4/1 -> Sum1/4
  Motor 3/1 -> Sum1/3
  Motor 2/1 -> Sum1/2
  Motor 1/1 -> Sum1/1
  CrossProduct(AXB)3/1(Out) -> Sum/4
  CrossProduct(AXB)2/1(Out) -> Sum/3
  CrossProduct(AXB)/1(Out) -> Sum/1
  Product4/1 -> CrossProduct(AXB)3/2(B)  "Thrust 4"
  Moment Arm4/1 -> CrossProduct(AXB)3/1(A)
  Product2/1 -> CrossProduct(AXB)2/2(B)  "Thrust 3"
  Moment Arm3/1 -> CrossProduct(AXB)2/1(A)
  Product1/1 -> CrossProduct(AXB)1/2(B)  "Thrust 2"
  Moment Arm2/1 -> CrossProduct(AXB)1/1(A)
  Product3/1 -> CrossProduct(AXB)/2(B)  "Thrust 1"
  Moment Arm1/1 -> CrossProduct(AXB)/1(A)
  Thrust Vector/1 -> Product8/2, Product6/2, Product5/2, Product7/2, Product4/2, Product2/2, Product1/2, Product3/2
  Demux/4 -> Product4/1
  Demux/3 -> Product2/1
  Demux/2 -> Product1/1
  Demux/1 -> Product3/1
  Thrust Magnitudes/1 -> Motor Thrust to Torques/1(Thrusts), Demux/1

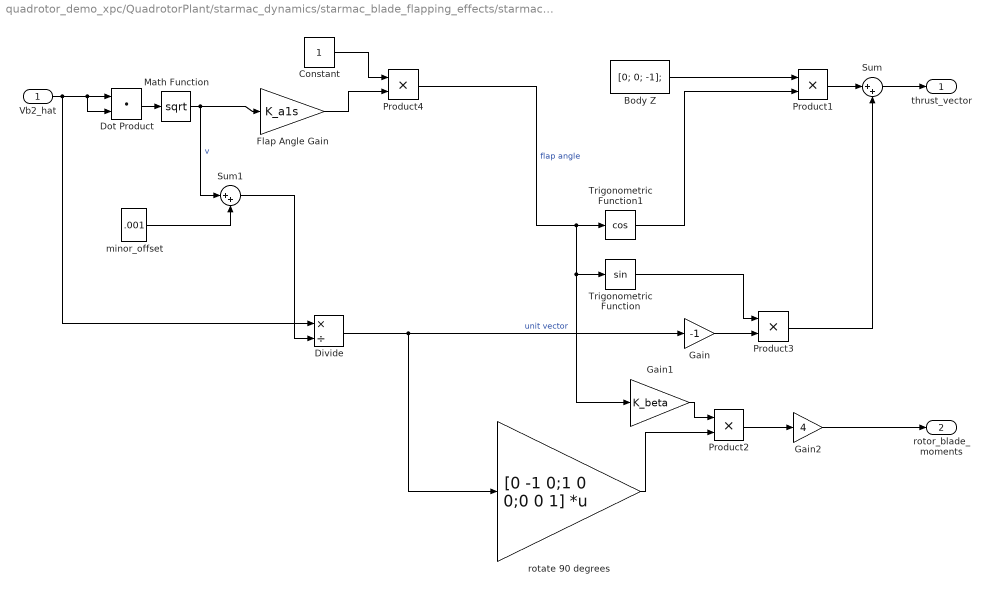
== system quadrotor_demo_xpc/QuadrotorPlant/starmac_dynamics/starmac_blade_flapping_effects/starmac_flapping_dynamics ==
  Vb2_hat : Inport  OutDataType=sfix(16)  OutScaling=2^0
  "Body Z " : Constant  Value=[0; 0; -1];  OutDataType=sfix(16)  OutScaling=2^0
  Constant : Constant  OutDataType=sfix(16)  OutScaling=2^0
  Divide : Product  Inputs=*/  OutDataType=sfix(16)  OutScaling=2^-10
  Dot Product : DotProduct  OutDataType=sfix(16)  OutScaling=2^-10  InputSameDT=on  OutDataTypeStr=Inherit: Inherit via internal rule
  Flap Angle Gain : Gain  Gain=K_a1s  ParameterDataType=sfix(16)  ParameterScaling=2^0  OutDataType=sfix(16)  OutScaling=2^0
  Gain : Gain  Gain=-1  ParameterDataType=sfix(16)  ParameterScaling=2^0  OutDataType=sfix(16)  OutScaling=2^0
  Gain1 : Gain  Gain=K_beta  ParameterDataType=sfix(16)  ParameterScaling=2^0  OutDataType=sfix(16)  OutScaling=2^0
  Gain2 : Gain  Gain=4  ParameterDataType=sfix(16)  ParameterScaling=2^0  OutDataType=sfix(16)  OutScaling=2^0
  Math Function : Math  Operator=sqrt  OutDataType=sfix(16)  OutScaling=2^0  SaturateOnIntegerOverflow=on
  Product{1..4} (4 alike) : Product  OutDataType=sfix(16)  OutScaling=2^0  RndMeth=Zero
  Sum : Sum  Inputs=|++  OutDataType=sfix(16)  OutScaling=2^0
  Sum1 : Sum  Inputs=|++  OutDataType=sfix(16)  OutScaling=2^0
  Trigonometric Function : Trigonometry
  Trigonometric Function1 : Trigonometry  Operator=cos
  minor_offset : Constant  Value=.001  OutDataType=sfix(16)  OutScaling=2^0
  rotate 90 degrees : Gain  Gain=[0 -1 0;1 0 0;0 0 1]  Multiplication=Matrix(K*u)  ParameterDataType=sfix(16)  ParameterScaling=2^0  OutDataType=sfix(16)  OutScaling=2^0
  thrust_vector : Outport  OutDataType=sfix(16)  OutScaling=2^0
  rotor_blade_moments : Outport  Port=2  OutDataType=sfix(16)  OutScaling=2^0
  wires:
  minor_offset/1 -> Sum1/2
  Sum1/1 -> Divide/2
  Divide/1 -> rotate 90 degrees/1, Gain/1  "unit vector"
  Product4/1 -> Trigonometric Function1/1, Trigonometric Function/1, Gain1/1  "flap angle"
  Vb2_hat/1 -> Divide/1, Dot Product/1, Dot Product/2
  Dot Product/1 -> Math Function/1
  Math Function/1 -> Sum1/1, Flap Angle Gain/1  "v"
  Trigonometric Function1/1 -> Product1/2
  Trigonometric Function/1 -> Product3/1
  Product3/1 -> Sum/2
  Gain/1 -> Product3/2
  Product1/1 -> Sum/1
  "Body Z "/1 -> Product1/1
  Sum/1 -> thrust_vector/1
  Gain2/1 -> rotor_blade_moments/1
  Product2/1 -> Gain2/1
  rotate 90 degrees/1 -> Product2/2
  Gain1/1 -> Product2/1
  Flap Angle Gain/1 -> Product4/2
  Constant/1 -> Product4/1

== system quadrotor_demo_xpc/QuadrotorPlant/starmac_dynamics/starmac_blade_flapping_effects/starmac_vertical_effect_dynamics ==
  motor_thrusts : Inport  OutDataType=sfix(16)  OutScaling=2^0
  v_body_relative : Inport  Port=2  OutDataType=sfix(16)  OutScaling=2^0
  Demux : Demux
  Mux : Mux
  starmac_motor_vertical_effect_dynamics{,1..3} (4 alike) : aero_sim_lib/starmac_motor_vertical_effect_dynamics  SystemSampleTime=-1  tau_motor=tau_motor  R=R  Alpha=Alpha  Vinf=Vinf  Vh=Vh  ToverTh=ToverTh
  thrust_multiplier : Outport  OutDataType=sfix(16)  OutScaling=2^0
  wires:
  motor_thrusts/1 -> Demux/1
  Mux/1 -> thrust_multiplier/1
  Demux/1 -> starmac_motor_vertical_effect_dynamics/1
  Demux/2 -> starmac_motor_vertical_effect_dynamics1/1
  Demux/3 -> starmac_motor_vertical_effect_dynamics2/1
  Demux/4 -> starmac_motor_vertical_effect_dynamics3/1
  starmac_motor_vertical_effect_dynamics/1 -> Mux/1
  starmac_motor_vertical_effect_dynamics1/1 -> Mux/2
  starmac_motor_vertical_effect_dynamics2/1 -> Mux/3
  starmac_motor_vertical_effect_dynamics3/1 -> Mux/4
  v_body_relative/1 -> starmac_motor_vertical_effect_dynamics2/2, starmac_motor_vertical_effect_dynamics3/2, starmac_motor_vertical_effect_dynamics1/2, starmac_motor_vertical_effect_dynamics/2

== system quadrotor_demo_xpc/QuadrotorPlant/starmac_dynamics/starmac_blade_flapping_effects/starmac_body_moments/CrossProduct(AXB) ==
  A : Inport  OutDataType=sfix(16)  OutScaling=2^0
  B : Inport  Port=2  OutDataType=sfix(16)  OutScaling=2^0
  Fcn : Fcn  Expr=u[2]*u[6]-u[3]*u[5]
  Fcn1 : Fcn  Expr=u[3]*u[4]-u[1]*u[6]
  Fcn2 : Fcn  Expr=u[1]*u[5]-u[2]*u[4]
  Mux : Mux  Inputs=2
  Mux1 : Mux  Inputs=3
  Out : Outport  OutDataType=sfix(16)  OutScaling=2^0
  wires:
  Mux1/1 -> Out/1
  Fcn2/1 -> Mux1/3
  Fcn1/1 -> Mux1/2
  Fcn/1 -> Mux1/1
  Mux/1 -> Fcn2/1, Fcn1/1, Fcn/1
  B/1 -> Mux/2
  A/1 -> Mux/1

== system quadrotor_demo_xpc/QuadrotorPlant/starmac_dynamics/starmac_blade_flapping_effects/starmac_body_moments/CrossProduct(AXB)1 ==
  A : Inport  OutDataType=sfix(16)  OutScaling=2^0
  B : Inport  Port=2  OutDataType=sfix(16)  OutScaling=2^0
  Fcn : Fcn  Expr=u[2]*u[6]-u[3]*u[5]
  Fcn1 : Fcn  Expr=u[3]*u[4]-u[1]*u[6]
  Fcn2 : Fcn  Expr=u[1]*u[5]-u[2]*u[4]
  Mux : Mux  Inputs=2
  Mux1 : Mux  Inputs=3
  Out : Outport  OutDataType=sfix(16)  OutScaling=2^0
  wires:
  A/1 -> Mux/1
  B/1 -> Mux/2
  Mux/1 -> Fcn/1, Fcn1/1, Fcn2/1
  Fcn/1 -> Mux1/1
  Fcn1/1 -> Mux1/2
  Fcn2/1 -> Mux1/3
  Mux1/1 -> Out/1

== system quadrotor_demo_xpc/QuadrotorPlant/starmac_dynamics/starmac_blade_flapping_effects/starmac_body_moments/CrossProduct(AXB)2 ==
  A : Inport  OutDataType=sfix(16)  OutScaling=2^0
  B : Inport  Port=2  OutDataType=sfix(16)  OutScaling=2^0
  Fcn : Fcn  Expr=u[2]*u[6]-u[3]*u[5]
  Fcn1 : Fcn  Expr=u[3]*u[4]-u[1]*u[6]
  Fcn2 : Fcn  Expr=u[1]*u[5]-u[2]*u[4]
  Mux : Mux  Inputs=2
  Mux1 : Mux  Inputs=3
  Out : Outport  OutDataType=sfix(16)  OutScaling=2^0
  wires:
  Mux1/1 -> Out/1
  Fcn2/1 -> Mux1/3
  Fcn1/1 -> Mux1/2
  Fcn/1 -> Mux1/1
  Mux/1 -> Fcn2/1, Fcn1/1, Fcn/1
  B/1 -> Mux/2
  A/1 -> Mux/1

== system quadrotor_demo_xpc/QuadrotorPlant/starmac_dynamics/starmac_blade_flapping_effects/starmac_body_moments/CrossProduct(AXB)3 ==
  A : Inport  OutDataType=sfix(16)  OutScaling=2^0
  B : Inport  Port=2  OutDataType=sfix(16)  OutScaling=2^0
  Fcn : Fcn  Expr=u[2]*u[6]-u[3]*u[5]
  Fcn1 : Fcn  Expr=u[3]*u[4]-u[1]*u[6]
  Fcn2 : Fcn  Expr=u[1]*u[5]-u[2]*u[4]
  Mux : Mux  Inputs=2
  Mux1 : Mux  Inputs=3
  Out : Outport  OutDataType=sfix(16)  OutScaling=2^0
  wires:
  A/1 -> Mux/1
  B/1 -> Mux/2
  Mux/1 -> Fcn/1, Fcn1/1, Fcn2/1
  Fcn/1 -> Mux1/1
  Fcn1/1 -> Mux1/2
  Fcn2/1 -> Mux1/3
  Mux1/1 -> Out/1

== system quadrotor_demo_xpc/QuadrotorPlant/starmac_dynamics/starmac_blade_flapping_effects/starmac_body_moments/Motor Thrust to Torques ==
  Thrusts : Inport  OutDataType=sfix(16)  OutScaling=2^0
  Demux : Demux
  Gain1 : Gain  Gain=K_torque  ParameterDataType=sfix(16)  ParameterScaling=2^0  OutDataType=sfix(16)  OutScaling=2^0
  torque 1 : Outport  OutDataType=sfix(16)  OutScaling=2^0
  torque 2 : Outport  Port=2  OutDataType=sfix(16)  OutScaling=2^0
  torque 3 : Outport  Port=3  OutDataType=sfix(16)  OutScaling=2^0
  torque 4 : Outport  Port=4  OutDataType=sfix(16)  OutScaling=2^0
  wires:
  Demux/4 -> torque 4/1
  Demux/3 -> torque 3/1
  Demux/2 -> torque 2/1
  Demux/1 -> torque 1/1
  Gain1/1 -> Demux/1
  Thrusts/1 -> Gain1/1
